simulink model "PD_Controller_mod"  (R2019b)
settings: Solver=VariableStepAuto  StartTime=0.0  StopTime=10  RelTol=1e-3
StopFcn:
  | Colors=hsv(5)';
  | for i=1:5
  | plot(out.tout,out.R_PD(:,i),'color',Colors(:,i),'LineWidth',1.5)
  | hold on
  | end
  | grid on
  | legend('Joint1','Joint2','Joint3','Joint4','Joint5')
  | title(['Response Vs Input of Joints Via PD Controller'])
  | xlabel('Time')
  | ylabel('Response')
libraries: simulink x5
(part 3 of 3)

== matlab function PD_Controller_mod/Robot_e_baba2 ==
  data: U input; q_ddot output; t input; tdot input
function q_ddot=fcn(U,t,tdot)

% t1=t(1);
t2=t(2);
t3=t(3);
t4=t(4);
t5=t(5);
% t6=t(6);

thetadot1=tdot(1);
thetadot2=tdot(2);
thetadot3=tdot(3);
thetadot4=tdot(4);
thetadot5=tdot(5);
% thetadot6=tdot(6);


M=[0.011148*cos(t5) + 4.3855*sin(t3) + 0.010268*cos(t5)*sin(t3) - 12.167*cos(t2)^2 - 1.6789*cos(t3)^2 - 0.0021796*cos(t4)^2 - 0.011148*cos(t2)^2*cos(t5) - 0.011148*cos(t3)^2*cos(t5) - 4.3855*cos(t2)^2*sin(t3) + 3.3578*cos(t2)^2*cos(t3)^2 + 0.0021796*cos(t2)^2*cos(t4)^2 - 0.00017962*cos(t2)^2*cos(t5)^2 + 0.0021796*cos(t3)^2*cos(t4)^2 - 0.00017962*cos(t3)^2*cos(t5)^2 + 0.00017962*cos(t4)^2*cos(t5)^2 - 0.0043592*cos(t2)^2*cos(t3)^2*cos(t4)^2 + 0.00035923*cos(t2)^2*cos(t3)^2*cos(t5)^2 - 0.00017962*cos(t2)^2*cos(t4)^2*cos(t5)^2 - 0.00017962*cos(t3)^2*cos(t4)^2*cos(t5)^2 - 0.010268*cos(t2)^2*cos(t5)*sin(t3) + 0.022296*cos(t2)^2*cos(t3)^2*cos(t5) - 4.3855*cos(t2)*cos(t3)*sin(t2) + 0.002*cos(t2)*cos(t4)*sin(t2) + 0.002*cos(t3)*cos(t4)*sin(t3) + 0.010268*cos(t3)*cos(t4)*sin(t5) - 0.004*cos(t2)*cos(t3)^2*cos(t4)*sin(t2) - 0.004*cos(t2)^2*cos(t3)*cos(t4)*sin(t3) - 0.010268*cos(t2)^2*cos(t3)*cos(t4)*sin(t5) + 0.00035923*cos(t2)^2*cos(t3)^2*cos(t4)^2*cos(t5)^2 - 0.010268*cos(t2)*cos(t3)*cos(t5)*sin(t2) - 3.3578*cos(t2)*cos(t3)*sin(t2)*sin(t3) + 0.011148*cos(t2)*cos(t4)*sin(t2)*sin(t5) + 0.011148*cos(t3)*cos(t4)*sin(t3)*sin(t5) + 0.0043592*cos(t2)*cos(t3)*cos(t4)^2*sin(t2)*sin(t3) - 0.00035923*cos(t2)*cos(t3)*cos(t5)^2*sin(t2)*sin(t3) - 0.022296*cos(t2)*cos(t3)^2*cos(t4)*sin(t2)*sin(t5) - 0.022296*cos(t2)^2*cos(t3)*cos(t4)*sin(t3)*sin(t5) - 0.022296*cos(t2)*cos(t3)*cos(t5)*sin(t2)*sin(t3) + 0.00035923*cos(t2)*cos(t4)*cos(t5)*sin(t2)*sin(t5) + 0.00035923*cos(t3)*cos(t4)*cos(t5)*sin(t3)*sin(t5) + 0.010268*cos(t2)*cos(t4)*sin(t2)*sin(t3)*sin(t5) - 0.00035923*cos(t2)*cos(t3)*cos(t4)^2*cos(t5)^2*sin(t2)*sin(t3) - 0.00071846*cos(t2)*cos(t3)^2*cos(t4)*cos(t5)*sin(t2)*sin(t5) - 0.00071846*cos(t2)^2*cos(t3)*cos(t4)*cos(t5)*sin(t3)*sin(t5) + 12.723, 0.11866*cos(t2) - 0.001*cos(t2)*cos(t3) + 0.001*sin(t2)*sin(t3) - 0.001*cos(t2)*sin(t3)*sin(t4) - 0.001*cos(t3)*sin(t2)*sin(t4) - 0.0051341*cos(t2)*sin(t4)*sin(t5) - 0.0021796*cos(t2)*cos(t3)*cos(t4)*sin(t4) + 0.0021796*cos(t4)*sin(t2)*sin(t3)*sin(t4) - 0.0055741*cos(t2)*sin(t3)*sin(t4)*sin(t5) - 0.0055741*cos(t3)*sin(t2)*sin(t4)*sin(t5) + 0.00017962*cos(t2)*cos(t3)*cos(t4)*cos(t5)^2*sin(t4) - 0.00017962*cos(t4)*cos(t5)^2*sin(t2)*sin(t3)*sin(t4) - 0.00017962*cos(t2)*cos(t5)*sin(t3)*sin(t4)*sin(t5) - 0.00017962*cos(t3)*cos(t5)*sin(t2)*sin(t4)*sin(t5), 0.001*sin(t2)*sin(t3) - 0.001*cos(t2)*cos(t3) - 0.001*cos(t2)*sin(t3)*sin(t4) - 0.001*cos(t3)*sin(t2)*sin(t4) - 0.0010449*sin(2.0*t4)*cos(t2)*cos(t3) + 0.0010449*sin(2.0*t4)*sin(t2)*sin(t3) + 0.000044904*cos(2.0*t5)*sin(2.0*t4)*cos(t2)*cos(t3) - 0.000044904*cos(2.0*t5)*sin(2.0*t4)*sin(t2)*sin(t3) - 0.000089808*sin(2.0*t5)*cos(t2)*sin(t3)*sin(t4) - 0.000089808*sin(2.0*t5)*cos(t3)*sin(t2)*sin(t4) - 0.0055741*cos(t2)*sin(t3)*sin(t4)*sin(t5) - 0.0055741*cos(t3)*sin(t2)*sin(t4)*sin(t5), 0.013*cos(t2)*sin(t3) + 0.013*cos(t3)*sin(t2) + 0.001*cos(t4)*sin(t2)*sin(t3) + 0.0051341*cos(t4)*sin(t2)*sin(t5) + 0.00017962*cos(t2)*sin(t3)*sin(t5)^2 + 0.00017962*cos(t3)*sin(t2)*sin(t5)^2 - 0.001*cos(t2)*cos(t3)*cos(t4) - 0.0055741*cos(t2)*cos(t3)*cos(t4)*sin(t5) + 0.0055741*cos(t4)*sin(t2)*sin(t3)*sin(t5) - 0.00017962*cos(t2)*cos(t3)*cos(t4)*cos(t5)*sin(t5) + 0.00017962*cos(t4)*cos(t5)*sin(t2)*sin(t3)*sin(t5), 1.0e-36*sin(t4)*(5.1341e+33*cos(t5)*sin(t2) - 1.7962e+32*cos(t2)*cos(t3) + 1.7962e+32*sin(t2)*sin(t3) + 5.5741e+33*cos(t5)*sin(t2)*sin(t3) - 5.5741e+33*cos(t2)*cos(t3)*cos(t5)), 0;
                                                                                                                                                                                                                                                                                                                                                                                                                                                                                                                                                                                                                                                                                                                                                                                                                                                                                                                                                                                                                                        0.11566*cos(t2) - 0.001*cos(t2)*cos(t3) + 0.001*sin(t2)*sin(t3) + 1.4349e-42*cos(2.0*t4)*cos(t2) - 0.001*cos(t2)*sin(t3)*sin(t4) - 0.001*cos(t3)*sin(t2)*sin(t4) - 0.0051341*cos(t2)*sin(t4)*sin(t5) + 3.5873e-43*cos(2.0*t3)*cos(2.0*t4)*cos(t2) + 3.5873e-43*cos(2.0*t4)*cos(2.0*t5)*cos(t2) + 3.5873e-43*cos(2.0*t4)*sin(2.0*t3)*sin(t2) - 3.5873e-43*cos(2.0*t5)*sin(2.0*t4)*sin(t2) - 0.0010449*sin(2.0*t4)*cos(t2)*cos(t3) + 0.0010449*sin(2.0*t4)*sin(t2)*sin(t3) + 0.000044904*cos(2.0*t5)*sin(2.0*t4)*cos(t2)*cos(t3) - 0.000044904*cos(2.0*t5)*sin(2.0*t4)*sin(t2)*sin(t3) - 0.000089808*sin(2.0*t5)*cos(t2)*sin(t3)*sin(t4) - 0.000089808*sin(2.0*t5)*cos(t3)*sin(t2)*sin(t4) - 0.0055741*cos(t2)*sin(t3)*sin(t4)*sin(t5) - 0.0055741*cos(t3)*sin(t2)*sin(t4)*sin(t5),                                                                                                                                                                                                                                                                                                                                                                                      0.011148*cos(t5) + 4.3855*sin(t3) + 0.010268*cos(t5)*sin(t3) + 0.0021796*cos(t4)^2 + 0.00017962*cos(t5)^2 - 0.00017962*cos(t4)^2*cos(t5)^2 + 0.010268*cos(t3)*cos(t4)*sin(t5) + 12.327,                                                                                                                                                                                                                                                                   0.0010449*cos(2.0*t4) + 0.000044904*cos(2.0*t5) + 0.011148*cos(t5) + 2.1928*sin(t3) + 0.0051341*cos(t5)*sin(t3) - 0.000044904*cos(2.0*t4)*cos(2.0*t5) + 1.5067e-40*cos(2.0*t4)*sin(t3) + 0.0051341*cos(t3)*cos(t4)*sin(t5) + 1.7641,                                                                                                                                                                                                                                                                                                                            -8.0e-36*sin(t4)*(1.1226e+31*sin(2.0*t5) + 6.9676e+32*sin(t5) + 6.4176e+32*sin(t3)*sin(t5) + 1.25e+32),                                                                   0.00017962*cos(t4) + 0.0055741*cos(t4)*cos(t5) + 0.0051341*cos(t3)*sin(t5) + 0.0051341*cos(t4)*cos(t5)*sin(t3), 0;
                                                                                                                                                                                                                                                                                                                                                                                                                                                                                                                                                                                                                                                                                                                                                                                                                                                                                                                                                                                                                                                                                                                                                                                                                                                                                                                   0.001*sin(t2)*sin(t3) - 0.001*cos(t2)*cos(t3) - 0.001*cos(t2)*sin(t3)*sin(t4) - 0.001*cos(t3)*sin(t2)*sin(t4) - 0.0010449*sin(2.0*t4)*cos(t2)*cos(t3) + 0.0010449*sin(2.0*t4)*sin(t2)*sin(t3) + 0.000044904*cos(2.0*t5)*sin(2.0*t4)*cos(t2)*cos(t3) - 0.000044904*cos(2.0*t5)*sin(2.0*t4)*sin(t2)*sin(t3) - 0.000089808*sin(2.0*t5)*cos(t2)*sin(t3)*sin(t4) - 0.000089808*sin(2.0*t5)*cos(t3)*sin(t2)*sin(t4) - 0.0055741*cos(t2)*sin(t3)*sin(t4)*sin(t5) - 0.0055741*cos(t3)*sin(t2)*sin(t4)*sin(t5),                                                                                                                                                                                                                                                                                                                                                                                    0.011148*cos(t5) + 2.1928*sin(t3) + 0.0051341*cos(t5)*sin(t3) + 0.0021796*cos(t4)^2 + 0.00017962*cos(t5)^2 - 0.00017962*cos(t4)^2*cos(t5)^2 + 0.0051341*cos(t3)*cos(t4)*sin(t5) + 1.7629,                                                                                                                                                                                                                                                                                                                                                                                     0.0010449*cos(2.0*t4) + 0.000044904*cos(2.0*t5) + 0.011148*cos(t5) - 0.000044904*cos(2.0*t4)*cos(2.0*t5) + 1.7641,                                                                                                                                                                                                                                                                                                                                                          -2.0e-36*sin(t4)*(4.4904e+31*sin(2.0*t5) + 2.7871e+33*sin(t5) + 5.0e+32),                                                                                                                                1.0e-36*cos(t4)*(5.5741e+33*cos(t5) + 1.7962e+32), 0;
                                                                                                                                                                                                                                                                                                                                                                                                                                                                                                                                                                                                                                                                                                                                                                                                                                                                                                                                                                                                                                                                                                                                                                                                                                                                                                                                                                                   0.01318*cos(t2)*sin(t3) + 0.01318*cos(t3)*sin(t2) + 0.001*cos(t4)*sin(t2)*sin(t3) + 0.0051341*cos(t4)*sin(t2)*sin(t5) - 0.00017962*cos(t2)*cos(t5)^2*sin(t3) - 0.00017962*cos(t3)*cos(t5)^2*sin(t2) - 0.001*cos(t2)*cos(t3)*cos(t4) - 0.0055741*cos(t2)*cos(t3)*cos(t4)*sin(t5) + 0.0055741*cos(t4)*sin(t2)*sin(t3)*sin(t5) - 0.00017962*cos(t2)*cos(t3)*cos(t4)*cos(t5)*sin(t5) + 0.00017962*cos(t4)*cos(t5)*sin(t2)*sin(t3)*sin(t5),                                                                                                                                                                                                                                                                                                                                                                                                                                                                      -8.0e-36*sin(t4)*(1.1226e+31*sin(2.0*t5) + 6.9676e+32*sin(t5) + 6.4176e+32*sin(t3)*sin(t5) + 1.25e+32),                                                                                                                                                                                                                                                                                                                                                                                                                             -8.0e-36*sin(t4)*(1.1226e+31*sin(2.0*t5) + 6.9676e+32*sin(t5) + 1.25e+32),                                                                                                                                                                                                                                                                                                                                                                                                      0.00017962*sin(t5)^2 + 0.013,                                                                                                                                                                                0, 0;
                                                                                                                                                                                                                                                                                                                                                                                                                                                                                                                                                                                                                                                                                                                                                                                                                                                                                                                                                                                                                                                                                                                                                                                                                                                                                                                                                                                                                                                                                                                                                                                                                                          2.4e-35*sin(t4)*(2.1392e+32*cos(t5)*sin(t2) - 7.484e+30*cos(t2)*cos(t3) + 7.484e+30*sin(t2)*sin(t3) + 2.3225e+32*cos(t5)*sin(t2)*sin(t3) - 2.3225e+32*cos(t2)*cos(t3)*cos(t5)),                                                                                                                                                                                                                                                                                                                                                                                                                                                              0.00017962*cos(t4) + 0.0055741*cos(t4)*cos(t5) + 0.0051341*cos(t3)*sin(t5) + 0.0051341*cos(t4)*cos(t5)*sin(t3),                                                                                                                                                                                                                                                                                                                                                                                                                                                      2.4e-35*cos(t4)*(2.3225e+32*cos(t5) + 7.484e+30),                                                                                                                                                                                                                                                                                                                                                                                                                                 0,                                                                                                                                                                       0.00017962, 0;
                                                                                                                                                                                                                                                                                                                                                                                                                                                                                                                                                                                                                                                                                                                                                                                                                                                                                                                                                                                                                                                                                                                                                                                                                                                                                                                                                                                                                                                                                                                                                                                                                                                                                                                                                                                                                       0,                                                                                                                                                                                                                                                                                                                                                                                                                                                                                                                                                                           0,                                                                                                                                                                                                                                                                                                                                                                                                                                                                                                     0,                                                                                                                                                                                                                                                                                                                                                                                                                                 0,                                                                                                                                                                                0, 0];




                                                                                                                                                                                                                                                                                                                                                                                                                                                                                                                                                                                                                                                                                                                                                                                                                                                                                                                                                                                                                                                                                                                                                                                                                                                                                                                                                                                                                                                                                                                                                                                                                                                                                                                                                                                                                   


C=[10.488*thetadot2*sin(2.0*t2) + 0.0010449*thetadot4*sin(2.0*t4) + 0.000044904*thetadot5*sin(2.0*t5) + 2.1928*thetadot3*cos(t3) - 0.0055741*thetadot5*sin(t5) - 4.3855*thetadot2*cos(2.0*t2)*cos(t3) - 2.1928*thetadot3*cos(2.0*t2)*cos(t3) + 4.3855*thetadot2*sin(2.0*t2)*sin(t3) + 2.1928*thetadot3*sin(2.0*t2)*sin(t3) + 0.0051341*thetadot3*cos(t3)*cos(t5) - 0.0051341*thetadot5*sin(t3)*sin(t5) - 1.678*thetadot2*cos(2.0*t2)*sin(2.0*t3) - 1.678*thetadot2*cos(2.0*t3)*sin(2.0*t2) - 1.678*thetadot3*cos(2.0*t2)*sin(2.0*t3) - 1.678*thetadot3*cos(2.0*t3)*sin(2.0*t2) - 0.000044904*thetadot4*cos(2.0*t5)*sin(2.0*t4) - 0.000044904*thetadot5*cos(2.0*t4)*sin(2.0*t5) + 0.010268*thetadot2*sin(2.0*t2)*cos(t5)*sin(t3) + 0.0051341*thetadot3*sin(2.0*t2)*cos(t5)*sin(t3) + 0.0051341*thetadot5*cos(2.0*t2)*sin(t3)*sin(t5) + 0.0051341*thetadot5*sin(2.0*t2)*cos(t3)*sin(t5) + 0.0010449*thetadot2*cos(2.0*t2)*cos(2.0*t4)*sin(2.0*t3) + 0.0010449*thetadot2*cos(2.0*t3)*cos(2.0*t4)*sin(2.0*t2) - 0.00013471*thetadot2*cos(2.0*t2)*cos(2.0*t5)*sin(2.0*t3) - 0.00013471*thetadot2*cos(2.0*t3)*cos(2.0*t5)*sin(2.0*t2) + 0.0010449*thetadot3*cos(2.0*t2)*cos(2.0*t4)*sin(2.0*t3) + 0.0010449*thetadot3*cos(2.0*t3)*cos(2.0*t4)*sin(2.0*t2) - 0.00013471*thetadot3*cos(2.0*t2)*cos(2.0*t5)*sin(2.0*t3) - 0.00013471*thetadot3*cos(2.0*t3)*cos(2.0*t5)*sin(2.0*t2) + 0.0010449*thetadot4*cos(2.0*t2)*cos(2.0*t3)*sin(2.0*t4) - 0.00013471*thetadot5*cos(2.0*t2)*cos(2.0*t3)*sin(2.0*t5) + 0.0051341*thetadot5*cos(t3)*cos(t4)*cos(t5) - 0.0010449*thetadot4*sin(2.0*t2)*sin(2.0*t3)*sin(2.0*t4) + 0.00013471*thetadot5*sin(2.0*t2)*sin(2.0*t3)*sin(2.0*t5) - 0.0051341*thetadot3*cos(t4)*sin(t3)*sin(t5) - 0.0051341*thetadot4*cos(t3)*sin(t4)*sin(t5) - 0.002*thetadot2*cos(2.0*t2)*cos(2.0*t3)*cos(t4) - 0.002*thetadot3*cos(2.0*t2)*cos(2.0*t3)*cos(t4) - 0.011148*thetadot2*cos(2.0*t2)*sin(2.0*t3)*cos(t5) - 0.011148*thetadot2*cos(2.0*t3)*sin(2.0*t2)*cos(t5) - 0.011148*thetadot3*cos(2.0*t2)*sin(2.0*t3)*cos(t5) - 0.011148*thetadot3*cos(2.0*t3)*sin(2.0*t2)*cos(t5) - 0.0055741*thetadot5*cos(2.0*t2)*cos(2.0*t3)*sin(t5) + 0.002*thetadot2*sin(2.0*t2)*sin(2.0*t3)*cos(t4) + 0.002*thetadot3*sin(2.0*t2)*sin(2.0*t3)*cos(t4) + 0.001*thetadot4*cos(2.0*t2)*sin(2.0*t3)*sin(t4) + 0.001*thetadot4*cos(2.0*t3)*sin(2.0*t2)*sin(t4) + 0.0055741*thetadot5*sin(2.0*t2)*sin(2.0*t3)*sin(t5) - 0.010268*thetadot2*cos(2.0*t2)*cos(t3)*cos(t5) - 0.0051341*thetadot3*cos(2.0*t2)*cos(t3)*cos(t5) - 0.0051341*thetadot4*sin(2.0*t2)*sin(t3)*sin(t4)*sin(t5) - 0.00017962*thetadot2*cos(2.0*t2)*cos(2.0*t3)*sin(2.0*t5)*cos(t4) - 0.00017962*thetadot3*cos(2.0*t2)*cos(2.0*t3)*sin(2.0*t5)*cos(t4) - 0.00017962*thetadot5*cos(2.0*t2)*cos(2.0*t5)*sin(2.0*t3)*cos(t4) - 0.00017962*thetadot5*cos(2.0*t3)*cos(2.0*t5)*sin(2.0*t2)*cos(t4) + 0.00017962*thetadot2*sin(2.0*t2)*sin(2.0*t3)*sin(2.0*t5)*cos(t4) + 0.00017962*thetadot3*sin(2.0*t2)*sin(2.0*t3)*sin(2.0*t5)*cos(t4) + 0.000089808*thetadot4*cos(2.0*t2)*sin(2.0*t3)*sin(2.0*t5)*sin(t4) + 0.000089808*thetadot4*cos(2.0*t3)*sin(2.0*t2)*sin(2.0*t5)*sin(t4) - 0.011148*thetadot2*cos(2.0*t2)*cos(2.0*t3)*cos(t4)*sin(t5) - 0.011148*thetadot3*cos(2.0*t2)*cos(2.0*t3)*cos(t4)*sin(t5) - 0.0055741*thetadot5*cos(2.0*t2)*sin(2.0*t3)*cos(t4)*cos(t5) - 0.0055741*thetadot5*cos(2.0*t3)*sin(2.0*t2)*cos(t4)*cos(t5) + 0.011148*thetadot2*sin(2.0*t2)*sin(2.0*t3)*cos(t4)*sin(t5) + 0.011148*thetadot3*sin(2.0*t2)*sin(2.0*t3)*cos(t4)*sin(t5) + 0.0055741*thetadot4*cos(2.0*t2)*sin(2.0*t3)*sin(t4)*sin(t5) + 0.0055741*thetadot4*cos(2.0*t3)*sin(2.0*t2)*sin(t4)*sin(t5) - 0.000044904*thetadot2*cos(2.0*t2)*cos(2.0*t4)*cos(2.0*t5)*sin(2.0*t3) - 0.000044904*thetadot2*cos(2.0*t3)*cos(2.0*t4)*cos(2.0*t5)*sin(2.0*t2) - 0.000044904*thetadot3*cos(2.0*t2)*cos(2.0*t4)*cos(2.0*t5)*sin(2.0*t3) - 0.000044904*thetadot3*cos(2.0*t3)*cos(2.0*t4)*cos(2.0*t5)*sin(2.0*t2) - 0.000044904*thetadot4*cos(2.0*t2)*cos(2.0*t3)*cos(2.0*t5)*sin(2.0*t4) - 0.000044904*thetadot5*cos(2.0*t2)*cos(2.0*t3)*cos(2.0*t4)*sin(2.0*t5) - 0.0051341*thetadot5*cos(2.0*t2)*cos(t3)*cos(t4)*cos(t5) + 0.000044904*thetadot4*cos(2.0*t5)*sin(2.0*t2)*sin(2.0*t3)*sin(2.0*t4) + 0.000044904*thetadot5*cos(2.0*t4)*sin(2.0*t2)*sin(2.0*t3)*sin(2.0*t5) + 0.010268*thetadot2*cos(2.0*t2)*cos(t4)*sin(t3)*sin(t5) + 0.010268*thetadot2*sin(2.0*t2)*cos(t3)*cos(t4)*sin(t5) + 0.0051341*thetadot3*cos(2.0*t2)*cos(t4)*sin(t3)*sin(t5) + 0.0051341*thetadot3*sin(2.0*t2)*cos(t3)*cos(t4)*sin(t5) + 0.0051341*thetadot4*cos(2.0*t2)*cos(t3)*sin(t4)*sin(t5) + 0.0051341*thetadot5*sin(2.0*t2)*cos(t4)*cos(t5)*sin(t3), 10.488*thetadot1*sin(2.0*t2) - 0.11866*thetadot2*sin(t2) - 4.3855*thetadot1*cos(2.0*t2)*cos(t3) + 4.3855*thetadot1*sin(2.0*t2)*sin(t3) + 0.01309*thetadot4*cos(t2)*cos(t3) + 0.001*thetadot2*cos(t2)*sin(t3) + 0.001*thetadot2*cos(t3)*sin(t2) + 0.002*thetadot3*cos(t2)*sin(t3) + 0.002*thetadot3*cos(t3)*sin(t2) - 0.01309*thetadot4*sin(t2)*sin(t3) - 1.678*thetadot1*cos(2.0*t2)*sin(2.0*t3) - 1.678*thetadot1*cos(2.0*t3)*sin(2.0*t2) + 0.010268*thetadot1*sin(2.0*t2)*cos(t5)*sin(t3) + 0.0010449*thetadot2*sin(2.0*t4)*cos(t2)*sin(t3) + 0.0010449*thetadot2*sin(2.0*t4)*cos(t3)*sin(t2) + 0.0020898*thetadot3*sin(2.0*t4)*cos(t2)*sin(t3) + 0.0020898*thetadot3*sin(2.0*t4)*cos(t3)*sin(t2) + 0.0020898*thetadot4*cos(2.0*t4)*sin(t2)*sin(t3) + 0.000089808*thetadot4*cos(2.0*t5)*sin(t2)*sin(t3) + 0.0010449*thetadot1*cos(2.0*t2)*cos(2.0*t4)*sin(2.0*t3) + 0.0010449*thetadot1*cos(2.0*t3)*cos(2.0*t4)*sin(2.0*t2) - 0.00013471*thetadot1*cos(2.0*t2)*cos(2.0*t5)*sin(2.0*t3) - 0.00013471*thetadot1*cos(2.0*t3)*cos(2.0*t5)*sin(2.0*t2) - 0.001*thetadot2*cos(t2)*cos(t3)*sin(t4) - 0.002*thetadot3*cos(t2)*cos(t3)*sin(t4) + 0.00017962*thetadot5*cos(t2)*sin(t3)*sin(t4) + 0.00017962*thetadot5*cos(t3)*sin(t2)*sin(t4) + 0.001*thetadot2*sin(t2)*sin(t3)*sin(t4) + 0.002*thetadot3*sin(t2)*sin(t3)*sin(t4) + 0.0051341*thetadot2*sin(t2)*sin(t4)*sin(t5) - 0.002*thetadot1*cos(2.0*t2)*cos(2.0*t3)*cos(t4) - 0.011148*thetadot1*cos(2.0*t2)*sin(2.0*t3)*cos(t5) - 0.011148*thetadot1*cos(2.0*t3)*sin(2.0*t2)*cos(t5) + 0.002*thetadot1*sin(2.0*t2)*sin(2.0*t3)*cos(t4) - 0.010268*thetadot1*cos(2.0*t2)*cos(t3)*cos(t5) - 0.0020898*thetadot4*cos(2.0*t4)*cos(t2)*cos(t3) - 0.000089808*thetadot4*cos(2.0*t5)*cos(t2)*cos(t3) + 0.000089808*thetadot2*sin(2.0*t5)*sin(t2)*sin(t3)*sin(t4) + 0.00017962*thetadot3*sin(2.0*t5)*sin(t2)*sin(t3)*sin(t4) - 0.00017962*thetadot1*cos(2.0*t2)*cos(2.0*t3)*sin(2.0*t5)*cos(t4) + 0.00017962*thetadot1*sin(2.0*t2)*sin(2.0*t3)*sin(2.0*t5)*cos(t4) - 0.0055741*thetadot2*cos(t2)*cos(t3)*sin(t4)*sin(t5) - 0.011148*thetadot3*cos(t2)*cos(t3)*sin(t4)*sin(t5) + 0.000089808*thetadot4*cos(2.0*t4)*cos(2.0*t5)*cos(t2)*cos(t3) + 0.0055741*thetadot2*sin(t2)*sin(t3)*sin(t4)*sin(t5) + 0.011148*thetadot3*sin(t2)*sin(t3)*sin(t4)*sin(t5) - 0.011148*thetadot1*cos(2.0*t2)*cos(2.0*t3)*cos(t4)*sin(t5) - 0.000044904*thetadot2*cos(2.0*t5)*sin(2.0*t4)*cos(t2)*sin(t3) - 0.000044904*thetadot2*cos(2.0*t5)*sin(2.0*t4)*cos(t3)*sin(t2) - 0.000089808*thetadot3*cos(2.0*t5)*sin(2.0*t4)*cos(t2)*sin(t3) - 0.000089808*thetadot3*cos(2.0*t5)*sin(2.0*t4)*cos(t3)*sin(t2) - 0.000089808*thetadot4*cos(2.0*t4)*cos(2.0*t5)*sin(t2)*sin(t3) - 0.000089808*thetadot5*sin(2.0*t4)*sin(2.0*t5)*cos(t2)*cos(t3) + 0.011148*thetadot1*sin(2.0*t2)*sin(2.0*t3)*cos(t4)*sin(t5) + 0.000089808*thetadot5*sin(2.0*t4)*sin(2.0*t5)*sin(t2)*sin(t3) - 0.000044904*thetadot1*cos(2.0*t2)*cos(2.0*t4)*cos(2.0*t5)*sin(2.0*t3) - 0.000044904*thetadot1*cos(2.0*t3)*cos(2.0*t4)*cos(2.0*t5)*sin(2.0*t2) + 0.010268*thetadot1*cos(2.0*t2)*cos(t4)*sin(t3)*sin(t5) + 0.010268*thetadot1*sin(2.0*t2)*cos(t3)*cos(t4)*sin(t5) - 0.000089808*thetadot2*sin(2.0*t5)*cos(t2)*cos(t3)*sin(t4) - 0.00017962*thetadot3*sin(2.0*t5)*cos(t2)*cos(t3)*sin(t4) - 0.00017962*thetadot5*cos(2.0*t5)*cos(t2)*sin(t3)*sin(t4) - 0.00017962*thetadot5*cos(2.0*t5)*cos(t3)*sin(t2)*sin(t4), 2.1928*thetadot1*cos(t3) - 2.1928*thetadot1*cos(2.0*t2)*cos(t3) + 2.1928*thetadot1*sin(2.0*t2)*sin(t3) + 0.0051341*thetadot1*cos(t3)*cos(t5) + 0.01309*thetadot4*cos(t2)*cos(t3) + 0.002*thetadot2*cos(t2)*sin(t3) + 0.002*thetadot2*cos(t3)*sin(t2) + 0.001*thetadot3*cos(t2)*sin(t3) + 0.001*thetadot3*cos(t3)*sin(t2) - 0.01309*thetadot4*sin(t2)*sin(t3) - 1.678*thetadot1*cos(2.0*t2)*sin(2.0*t3) - 1.678*thetadot1*cos(2.0*t3)*sin(2.0*t2) + 0.0051341*thetadot1*sin(2.0*t2)*cos(t5)*sin(t3) + 0.0020898*thetadot2*sin(2.0*t4)*cos(t2)*sin(t3) + 0.0020898*thetadot2*sin(2.0*t4)*cos(t3)*sin(t2) + 0.0010449*thetadot3*sin(2.0*t4)*cos(t2)*sin(t3) + 0.0010449*thetadot3*sin(2.0*t4)*cos(t3)*sin(t2) + 0.0020898*thetadot4*cos(2.0*t4)*sin(t2)*sin(t3) + 0.000089808*thetadot4*cos(2.0*t5)*sin(t2)*sin(t3) + 0.0010449*thetadot1*cos(2.0*t2)*cos(2.0*t4)*sin(2.0*t3) + 0.0010449*thetadot1*cos(2.0*t3)*cos(2.0*t4)*sin(2.0*t2) - 0.00013471*thetadot1*cos(2.0*t2)*cos(2.0*t5)*sin(2.0*t3) - 0.00013471*thetadot1*cos(2.0*t3)*cos(2.0*t5)*sin(2.0*t2) - 0.002*thetadot2*cos(t2)*cos(t3)*sin(t4) - 0.001*thetadot3*cos(t2)*cos(t3)*sin(t4) - 0.0051341*thetadot1*cos(t4)*sin(t3)*sin(t5) + 0.00017962*thetadot5*cos(t2)*sin(t3)*sin(t4) + 0.00017962*thetadot5*cos(t3)*sin(t2)*sin(t4) + 0.002*thetadot2*sin(t2)*sin(t3)*sin(t4) + 0.001*thetadot3*sin(t2)*sin(t3)*sin(t4) - 0.002*thetadot1*cos(2.0*t2)*cos(2.0*t3)*cos(t4) - 0.011148*thetadot1*cos(2.0*t2)*sin(2.0*t3)*cos(t5) - 0.011148*thetadot1*cos(2.0*t3)*sin(2.0*t2)*cos(t5) + 0.002*thetadot1*sin(2.0*t2)*sin(2.0*t3)*cos(t4) - 0.0051341*thetadot1*cos(2.0*t2)*cos(t3)*cos(t5) - 0.0020898*thetadot4*cos(2.0*t4)*cos(t2)*cos(t3) - 0.000089808*thetadot4*cos(2.0*t5)*cos(t2)*cos(t3) + 0.00017962*thetadot2*sin(2.0*t5)*sin(t2)*sin(t3)*sin(t4) + 0.000089808*thetadot3*sin(2.0*t5)*sin(t2)*sin(t3)*sin(t4) - 0.00017962*thetadot1*cos(2.0*t2)*cos(2.0*t3)*sin(2.0*t5)*cos(t4) + 0.00017962*thetadot1*sin(2.0*t2)*sin(2.0*t3)*sin(2.0*t5)*cos(t4) - 0.011148*thetadot2*cos(t2)*cos(t3)*sin(t4)*sin(t5) - 0.0055741*thetadot3*cos(t2)*cos(t3)*sin(t4)*sin(t5) + 0.000089808*thetadot4*cos(2.0*t4)*cos(2.0*t5)*cos(t2)*cos(t3) + 0.011148*thetadot2*sin(t2)*sin(t3)*sin(t4)*sin(t5) + 0.0055741*thetadot3*sin(t2)*sin(t3)*sin(t4)*sin(t5) - 0.011148*thetadot1*cos(2.0*t2)*cos(2.0*t3)*cos(t4)*sin(t5) - 0.000089808*thetadot2*cos(2.0*t5)*sin(2.0*t4)*cos(t2)*sin(t3) - 0.000089808*thetadot2*cos(2.0*t5)*sin(2.0*t4)*cos(t3)*sin(t2) - 0.000044904*thetadot3*cos(2.0*t5)*sin(2.0*t4)*cos(t2)*sin(t3) - 0.000044904*thetadot3*cos(2.0*t5)*sin(2.0*t4)*cos(t3)*sin(t2) - 0.000089808*thetadot4*cos(2.0*t4)*cos(2.0*t5)*sin(t2)*sin(t3) - 0.000089808*thetadot5*sin(2.0*t4)*sin(2.0*t5)*cos(t2)*cos(t3) + 0.011148*thetadot1*sin(2.0*t2)*sin(2.0*t3)*cos(t4)*sin(t5) + 0.000089808*thetadot5*sin(2.0*t4)*sin(2.0*t5)*sin(t2)*sin(t3) - 0.000044904*thetadot1*cos(2.0*t2)*cos(2.0*t4)*cos(2.0*t5)*sin(2.0*t3) - 0.000044904*thetadot1*cos(2.0*t3)*cos(2.0*t4)*cos(2.0*t5)*sin(2.0*t2) + 0.0051341*thetadot1*cos(2.0*t2)*cos(t4)*sin(t3)*sin(t5) + 0.0051341*thetadot1*sin(2.0*t2)*cos(t3)*cos(t4)*sin(t5) - 0.00017962*thetadot2*sin(2.0*t5)*cos(t2)*cos(t3)*sin(t4) - 0.000089808*thetadot3*sin(2.0*t5)*cos(t2)*cos(t3)*sin(t4) - 0.00017962*thetadot5*cos(2.0*t5)*cos(t2)*sin(t3)*sin(t4) - 0.00017962*thetadot5*cos(2.0*t5)*cos(t3)*sin(t2)*sin(t4), 0.0010449*thetadot1*sin(2.0*t4) + 0.01309*thetadot2*cos(t2)*cos(t3) + 0.01309*thetadot3*cos(t2)*cos(t3) - 0.01309*thetadot2*sin(t2)*sin(t3) - 0.01309*thetadot3*sin(t2)*sin(t3) - 0.000044904*thetadot1*cos(2.0*t5)*sin(2.0*t4) + 0.0020898*thetadot2*cos(2.0*t4)*sin(t2)*sin(t3) + 0.000089808*thetadot2*cos(2.0*t5)*sin(t2)*sin(t3) + 0.0020898*thetadot3*cos(2.0*t4)*sin(t2)*sin(t3) + 0.000089808*thetadot3*cos(2.0*t5)*sin(t2)*sin(t3) + 0.00017962*thetadot5*sin(2.0*t5)*cos(t2)*sin(t3) + 0.00017962*thetadot5*sin(2.0*t5)*cos(t3)*sin(t2) + 0.0010449*thetadot1*cos(2.0*t2)*cos(2.0*t3)*sin(2.0*t4) - 0.00017962*thetadot5*cos(t2)*cos(t3)*cos(t4) - 0.0010449*thetadot1*sin(2.0*t2)*sin(2.0*t3)*sin(2.0*t4) + 0.001*thetadot4*cos(t2)*cos(t3)*sin(t4) + 0.010268*thetadot5*cos(t4)*cos(t5)*sin(t2) - 0.0051341*thetadot1*cos(t3)*sin(t4)*sin(t5) + 0.00017962*thetadot5*cos(t4)*sin(t2)*sin(t3) - 0.001*thetadot4*sin(t2)*sin(t3)*sin(t4) - 0.0051341*thetadot4*sin(t2)*sin(t4)*sin(t5) + 0.001*thetadot1*cos(2.0*t2)*sin(2.0*t3)*sin(t4) + 0.001*thetadot1*cos(2.0*t3)*sin(2.0*t2)*sin(t4) - 0.0020898*thetadot2*cos(2.0*t4)*cos(t2)*cos(t3) - 0.000089808*thetadot2*cos(2.0*t5)*cos(t2)*cos(t3) - 0.0020898*thetadot3*cos(2.0*t4)*cos(t2)*cos(t3) - 0.000089808*thetadot3*cos(2.0*t5)*cos(t2)*cos(t3) - 0.0051341*thetadot1*sin(2.0*t2)*sin(t3)*sin(t4)*sin(t5) - 0.000089808*thetadot4*sin(2.0*t5)*sin(t2)*sin(t3)*sin(t4) - 0.011148*thetadot5*cos(t2)*cos(t3)*cos(t4)*cos(t5) + 0.000089808*thetadot1*cos(2.0*t2)*sin(2.0*t3)*sin(2.0*t5)*sin(t4) + 0.000089808*thetadot1*cos(2.0*t3)*sin(2.0*t2)*sin(2.0*t5)*sin(t4) + 0.0055741*thetadot4*cos(t2)*cos(t3)*sin(t4)*sin(t5) + 0.011148*thetadot5*cos(t4)*cos(t5)*sin(t2)*sin(t3) + 0.000089808*thetadot2*cos(2.0*t4)*cos(2.0*t5)*cos(t2)*cos(t3) + 0.000089808*thetadot3*cos(2.0*t4)*cos(2.0*t5)*cos(t2)*cos(t3) - 0.0055741*thetadot4*sin(t2)*sin(t3)*sin(t4)*sin(t5) - 0.000089808*thetadot2*cos(2.0*t4)*cos(2.0*t5)*sin(t2)*sin(t3) - 0.000089808*thetadot3*cos(2.0*t4)*cos(2.0*t5)*sin(t2)*sin(t3) + 0.0055741*thetadot1*cos(2.0*t2)*sin(2.0*t3)*sin(t4)*sin(t5) + 0.0055741*thetadot1*cos(2.0*t3)*sin(2.0*t2)*sin(t4)*sin(t5) - 0.000044904*thetadot1*cos(2.0*t2)*cos(2.0*t3)*cos(2.0*t5)*sin(2.0*t4) - 0.00017962*thetadot5*cos(2.0*t5)*cos(t2)*cos(t3)*cos(t4) + 0.000044904*thetadot1*cos(2.0*t5)*sin(2.0*t2)*sin(2.0*t3)*sin(2.0*t4) + 0.0051341*thetadot1*cos(2.0*t2)*cos(t3)*sin(t4)*sin(t5) + 0.000089808*thetadot4*sin(2.0*t5)*cos(t2)*cos(t3)*sin(t4) + 0.00017962*thetadot5*cos(2.0*t5)*cos(t4)*sin(t2)*sin(t3), 0.000044904*thetadot1*sin(2.0*t5) - 0.0055741*thetadot1*sin(t5) - 0.0051341*thetadot1*sin(t3)*sin(t5) - 0.000044904*thetadot1*cos(2.0*t4)*sin(2.0*t5) + 0.0051341*thetadot1*cos(2.0*t2)*sin(t3)*sin(t5) + 0.0051341*thetadot1*sin(2.0*t2)*cos(t3)*sin(t5) + 0.00017962*thetadot4*sin(2.0*t5)*cos(t2)*sin(t3) + 0.00017962*thetadot4*sin(2.0*t5)*cos(t3)*sin(t2) - 0.00013471*thetadot1*cos(2.0*t2)*cos(2.0*t3)*sin(2.0*t5) + 0.0051341*thetadot1*cos(t3)*cos(t4)*cos(t5) - 0.00017962*thetadot4*cos(t2)*cos(t3)*cos(t4) + 0.00013471*thetadot1*sin(2.0*t2)*sin(2.0*t3)*sin(2.0*t5) + 0.010268*thetadot4*cos(t4)*cos(t5)*sin(t2) + 0.00017962*thetadot2*cos(t2)*sin(t3)*sin(t4) + 0.00017962*thetadot2*cos(t3)*sin(t2)*sin(t4) + 0.00017962*thetadot3*cos(t2)*sin(t3)*sin(t4) + 0.00017962*thetadot3*cos(t3)*sin(t2)*sin(t4) + 0.00017962*thetadot4*cos(t4)*sin(t2)*sin(t3) - 0.0051341*thetadot5*sin(t2)*sin(t4)*sin(t5) - 0.0055741*thetadot1*cos(2.0*t2)*cos(2.0*t3)*sin(t5) + 0.0055741*thetadot1*sin(2.0*t2)*sin(2.0*t3)*sin(t5) - 0.00017962*thetadot1*cos(2.0*t2)*cos(2.0*t5)*sin(2.0*t3)*cos(t4) - 0.00017962*thetadot1*cos(2.0*t3)*cos(2.0*t5)*sin(2.0*t2)*cos(t4) - 0.011148*thetadot4*cos(t2)*cos(t3)*cos(t4)*cos(t5) + 0.011148*thetadot4*cos(t4)*cos(t5)*sin(t2)*sin(t3) + 0.0055741*thetadot5*cos(t2)*cos(t3)*sin(t4)*sin(t5) - 0.0055741*thetadot5*sin(t2)*sin(t3)*sin(t4)*sin(t5) - 0.0055741*thetadot1*cos(2.0*t2)*sin(2.0*t3)*cos(t4)*cos(t5) - 0.0055741*thetadot1*cos(2.0*t3)*sin(2.0*t2)*cos(t4)*cos(t5) - 0.000089808*thetadot2*sin(2.0*t4)*sin(2.0*t5)*cos(t2)*cos(t3) - 0.000089808*thetadot3*sin(2.0*t4)*sin(2.0*t5)*cos(t2)*cos(t3) + 0.000089808*thetadot2*sin(2.0*t4)*sin(2.0*t5)*sin(t2)*sin(t3) + 0.000089808*thetadot3*sin(2.0*t4)*sin(2.0*t5)*sin(t2)*sin(t3) - 0.000044904*thetadot1*cos(2.0*t2)*cos(2.0*t3)*cos(2.0*t4)*sin(2.0*t5) - 0.0051341*thetadot1*cos(2.0*t2)*cos(t3)*cos(t4)*cos(t5) - 0.00017962*thetadot4*cos(2.0*t5)*cos(t2)*cos(t3)*cos(t4) + 0.000044904*thetadot1*cos(2.0*t4)*sin(2.0*t2)*sin(2.0*t3)*sin(2.0*t5) + 0.0051341*thetadot1*sin(2.0*t2)*cos(t4)*cos(t5)*sin(t3) - 0.00017962*thetadot2*cos(2.0*t5)*cos(t2)*sin(t3)*sin(t4) - 0.00017962*thetadot2*cos(2.0*t5)*cos(t3)*sin(t2)*sin(t4) - 0.00017962*thetadot3*cos(2.0*t5)*cos(t2)*sin(t3)*sin(t4) - 0.00017962*thetadot3*cos(2.0*t5)*cos(t3)*sin(t2)*sin(t4) + 0.00017962*thetadot4*cos(2.0*t5)*cos(t4)*sin(t2)*sin(t3), 0;
                                                                                                                                                                                                                                                                                                                                                                                                                                                                                                                                                                                                                                                                                                                                                                                                                                                                                                                                                                                                                                                                                                                                                                                                                                                                                                                                                                                                                                                                                                                                                                                                                                                                                                                                                                                                                                                                                                                                                                                                                        0.003*thetadot2*sin(t2) - 5.2441*thetadot1*sin(2.0*t2) + 2.1928*thetadot1*cos(2.0*t2)*cos(t3) - 2.1928*thetadot1*sin(2.0*t2)*sin(t3) - 0.01309*thetadot4*cos(t2)*cos(t3) + 0.01309*thetadot4*sin(t2)*sin(t3) + 0.83898*thetadot1*cos(2.0*t2)*sin(2.0*t3) + 0.83898*thetadot1*cos(2.0*t3)*sin(2.0*t2) - 0.0051341*thetadot1*sin(2.0*t2)*cos(t5)*sin(t3) + 0.0020898*thetadot4*cos(2.0*t4)*sin(t2)*sin(t3) - 0.000089808*thetadot4*cos(2.0*t5)*sin(t2)*sin(t3) - 0.00052245*thetadot1*cos(2.0*t2)*cos(2.0*t4)*sin(2.0*t3) - 0.00052245*thetadot1*cos(2.0*t3)*cos(2.0*t4)*sin(2.0*t2) + 0.000067356*thetadot1*cos(2.0*t2)*cos(2.0*t5)*sin(2.0*t3) + 0.000067356*thetadot1*cos(2.0*t3)*cos(2.0*t5)*sin(2.0*t2) - 0.002*thetadot4*cos(t2)*cos(t4)*sin(t3) - 0.002*thetadot4*cos(t3)*cos(t4)*sin(t2) - 0.010268*thetadot4*cos(t2)*cos(t4)*sin(t5) - 0.010268*thetadot5*cos(t2)*cos(t5)*sin(t4) - 0.00017962*thetadot5*cos(t2)*sin(t3)*sin(t4) - 0.00017962*thetadot5*cos(t3)*sin(t2)*sin(t4) + 0.001*thetadot1*cos(2.0*t2)*cos(2.0*t3)*cos(t4) + 0.0055741*thetadot1*cos(2.0*t2)*sin(2.0*t3)*cos(t5) + 0.0055741*thetadot1*cos(2.0*t3)*sin(2.0*t2)*cos(t5) - 0.001*thetadot1*sin(2.0*t2)*sin(2.0*t3)*cos(t4) + 0.0051341*thetadot1*cos(2.0*t2)*cos(t3)*cos(t5) - 0.0020898*thetadot4*cos(2.0*t4)*cos(t2)*cos(t3) + 0.000089808*thetadot4*cos(2.0*t5)*cos(t2)*cos(t3) + 0.000089808*thetadot1*cos(2.0*t2)*cos(2.0*t3)*sin(2.0*t5)*cos(t4) - 0.000089808*thetadot1*sin(2.0*t2)*sin(2.0*t3)*sin(2.0*t5)*cos(t4) - 0.011148*thetadot4*cos(t2)*cos(t4)*sin(t3)*sin(t5) - 0.011148*thetadot4*cos(t3)*cos(t4)*sin(t2)*sin(t5) - 0.011148*thetadot5*cos(t2)*cos(t5)*sin(t3)*sin(t4) - 0.011148*thetadot5*cos(t3)*cos(t5)*sin(t2)*sin(t4) + 0.000089808*thetadot4*cos(2.0*t4)*cos(2.0*t5)*cos(t2)*cos(t3) + 0.0055741*thetadot1*cos(2.0*t2)*cos(2.0*t3)*cos(t4)*sin(t5) - 0.000089808*thetadot4*cos(2.0*t4)*cos(2.0*t5)*sin(t2)*sin(t3) - 0.000089808*thetadot5*sin(2.0*t4)*sin(2.0*t5)*cos(t2)*cos(t3) - 0.0055741*thetadot1*sin(2.0*t2)*sin(2.0*t3)*cos(t4)*sin(t5) + 0.000089808*thetadot5*sin(2.0*t4)*sin(2.0*t5)*sin(t2)*sin(t3) + 0.000022452*thetadot1*cos(2.0*t2)*cos(2.0*t4)*cos(2.0*t5)*sin(2.0*t3) + 0.000022452*thetadot1*cos(2.0*t3)*cos(2.0*t4)*cos(2.0*t5)*sin(2.0*t2) - 0.0051341*thetadot1*cos(2.0*t2)*cos(t4)*sin(t3)*sin(t5) - 0.0051341*thetadot1*sin(2.0*t2)*cos(t3)*cos(t4)*sin(t5) - 0.00017962*thetadot4*sin(2.0*t5)*cos(t2)*cos(t4)*sin(t3) - 0.00017962*thetadot4*sin(2.0*t5)*cos(t3)*cos(t4)*sin(t2) - 0.00017962*thetadot5*cos(2.0*t5)*cos(t2)*sin(t3)*sin(t4) - 0.00017962*thetadot5*cos(2.0*t5)*cos(t3)*sin(t2)*sin(t4),                                                                                                                                                                                                                                                                                                                                                                                                                                                                                                                                                                                                                                                                                                                                                                                                                                                                                                                                                                                                                                                                                                                                                                                                                                                                                                                                                                                                                                                                                                                                                                                                                                                                                                                                                                                                                                                                                                                                                                                                                                                                                                                                                                                                                                                                                                                                                                                                                                                                                                                                                                                                                                                                                                                                                                                                                                                                                                                                   4.3855*thetadot3*cos(t3) - 0.000089808*thetadot5*sin(2.0*t5) - 0.0020898*thetadot4*sin(2.0*t4) + 0.003*thetadot1*sin(t2) - 0.011148*thetadot5*sin(t5) + 0.010268*thetadot3*cos(t3)*cos(t5) - 0.010268*thetadot5*sin(t3)*sin(t5) + 0.000089808*thetadot4*cos(2.0*t5)*sin(2.0*t4) + 0.000089808*thetadot5*cos(2.0*t4)*sin(2.0*t5) + 0.010268*thetadot5*cos(t3)*cos(t4)*cos(t5) - 0.010268*thetadot3*cos(t4)*sin(t3)*sin(t5) - 0.010268*thetadot4*cos(t3)*sin(t4)*sin(t5),                                                                                                                                                                                                                                                                                                                                                                                                                                                                                                                                                                                                                                                                                                                                                                                                                                                                                                                                                                                                                                                                                                                                                                                                                                                                                                                                                                                                                                                                                                                                                                                                                                                                                                                                                                                                                                                                                                                                                                                                                                                                                                                                                                                                                                                                                                                                                                                                                                                                                                                                                                                                                                                                                                                                                                                                                                                        4.3855*thetadot2*cos(t3) - 0.000089808*thetadot5*sin(2.0*t5) - 0.0020898*thetadot4*sin(2.0*t4) + 2.1928*thetadot3*cos(t3) - 0.011148*thetadot5*sin(t5) + 0.010268*thetadot2*cos(t3)*cos(t5) + 0.0051341*thetadot3*cos(t3)*cos(t5) - 0.010268*thetadot5*sin(t3)*sin(t5) + 0.000089808*thetadot4*cos(2.0*t5)*sin(2.0*t4) + 0.000089808*thetadot5*cos(2.0*t4)*sin(2.0*t5) + 0.010268*thetadot5*cos(t3)*cos(t4)*cos(t5) - 0.010268*thetadot2*cos(t4)*sin(t3)*sin(t5) - 0.0051341*thetadot3*cos(t4)*sin(t3)*sin(t5) - 0.010268*thetadot4*cos(t3)*sin(t4)*sin(t5),                                                                                                                                                                                                                                                                                                                                                                                                                                                                                                                                                                                                                                                                                                                                                                                                                                                                                                                                                                                                                                                                                                                                                                                                                                                                                                                                                                     0.011*thetadot1*sin(t2)*sin(t3) - 0.0021796*thetadot3*sin(2.0*t4) - 0.001*thetadot4*cos(t4) - 0.011*thetadot1*cos(t2)*cos(t3) - 0.0055741*thetadot4*cos(t4)*sin(t5) - 0.011148*thetadot5*cos(t5)*sin(t4) - 0.0021796*thetadot2*sin(2.0*t4) - 0.00035923*thetadot5*cos(t5)^2*sin(t4) - 0.002*thetadot1*cos(t2)*cos(t4)*sin(t3) - 0.002*thetadot1*cos(t3)*cos(t4)*sin(t2) - 0.010268*thetadot1*cos(t2)*cos(t4)*sin(t5) - 0.00017962*thetadot4*cos(t4)*cos(t5)*sin(t5) - 0.010268*thetadot2*cos(t3)*sin(t4)*sin(t5) - 0.010268*thetadot3*cos(t3)*sin(t4)*sin(t5) - 0.0051341*thetadot4*cos(t4)*sin(t3)*sin(t5) - 0.010268*thetadot5*cos(t5)*sin(t3)*sin(t4) - 0.0043592*thetadot1*cos(t2)*cos(t3)*cos(t4)^2 + 0.00035923*thetadot2*cos(t4)*cos(t5)^2*sin(t4) + 0.00035923*thetadot3*cos(t4)*cos(t5)^2*sin(t4) + 0.0043592*thetadot1*cos(t4)^2*sin(t2)*sin(t3) - 0.00035923*thetadot1*cos(t4)^2*cos(t5)^2*sin(t2)*sin(t3) - 0.011148*thetadot1*cos(t2)*cos(t4)*sin(t3)*sin(t5) - 0.011148*thetadot1*cos(t3)*cos(t4)*sin(t2)*sin(t5) + 0.00035923*thetadot1*cos(t2)*cos(t3)*cos(t4)^2*cos(t5)^2 - 0.00035923*thetadot1*cos(t2)*cos(t4)*cos(t5)*sin(t3)*sin(t5) - 0.00035923*thetadot1*cos(t3)*cos(t4)*cos(t5)*sin(t2)*sin(t5),                                                                                                                                                                                                                                                                                                                                                                                                                                                                                                                                                                                                                                                                                                                                                                                                                                                                                                                                                                                                                                                                                                                                                                                                                                                                                                                                                    0.0051341*thetadot5*cos(t3)*cos(t5) - 0.00017962*thetadot3*sin(2.0*t5) - 0.011148*thetadot2*sin(t5) - 0.011148*thetadot3*sin(t5) - 0.00017962*thetadot2*sin(2.0*t5) - 0.011148*thetadot4*cos(t5)*sin(t4) - 0.0055741*thetadot5*cos(t4)*sin(t5) - 0.010268*thetadot2*sin(t3)*sin(t5) - 0.010268*thetadot3*sin(t3)*sin(t5) - 0.00035923*thetadot4*cos(t5)^2*sin(t4) + 0.010268*thetadot2*cos(t3)*cos(t4)*cos(t5) + 0.010268*thetadot3*cos(t3)*cos(t4)*cos(t5) - 0.010268*thetadot1*cos(t2)*cos(t5)*sin(t4) - 0.010268*thetadot4*cos(t5)*sin(t3)*sin(t4) - 0.0051341*thetadot5*cos(t4)*sin(t3)*sin(t5) + 0.00035923*thetadot2*cos(t4)^2*cos(t5)*sin(t5) + 0.00035923*thetadot3*cos(t4)^2*cos(t5)*sin(t5) - 0.011148*thetadot1*cos(t2)*cos(t5)*sin(t3)*sin(t4) - 0.011148*thetadot1*cos(t3)*cos(t5)*sin(t2)*sin(t4) - 0.00035923*thetadot1*cos(t2)*cos(t5)^2*sin(t3)*sin(t4) - 0.00035923*thetadot1*cos(t3)*cos(t5)^2*sin(t2)*sin(t4) - 0.00035923*thetadot1*cos(t2)*cos(t3)*cos(t4)*cos(t5)*sin(t4)*sin(t5) + 0.00035923*thetadot1*cos(t4)*cos(t5)*sin(t2)*sin(t3)*sin(t4)*sin(t5), 0;
                                                                                                                                                                                                                                                                                                                                                                                                                                                                                                                                                                                                                                                                                                                                                                                                                                                                                                                                                                                                                                                                                                                                                                                                                                                                                                                                                                                                                                                                                                                                                                                                                                                                                                                                                                                                                                                                                                                                                                                                                                                                  1.0964*thetadot1*cos(2.0*t2)*cos(t3) - 1.0964*thetadot1*cos(t3) - 1.0964*thetadot1*sin(2.0*t2)*sin(t3) - 0.002567*thetadot1*cos(t3)*cos(t5) - 0.01309*thetadot4*cos(t2)*cos(t3) + 0.01309*thetadot4*sin(t2)*sin(t3) + 0.83898*thetadot1*cos(2.0*t2)*sin(2.0*t3) + 0.83898*thetadot1*cos(2.0*t3)*sin(2.0*t2) - 0.002567*thetadot1*sin(2.0*t2)*cos(t5)*sin(t3) + 0.0020898*thetadot4*cos(2.0*t4)*sin(t2)*sin(t3) - 0.000089808*thetadot4*cos(2.0*t5)*sin(t2)*sin(t3) - 0.00052245*thetadot1*cos(2.0*t2)*cos(2.0*t4)*sin(2.0*t3) - 0.00052245*thetadot1*cos(2.0*t3)*cos(2.0*t4)*sin(2.0*t2) + 0.000067356*thetadot1*cos(2.0*t2)*cos(2.0*t5)*sin(2.0*t3) + 0.000067356*thetadot1*cos(2.0*t3)*cos(2.0*t5)*sin(2.0*t2) - 0.002*thetadot4*cos(t2)*cos(t4)*sin(t3) - 0.002*thetadot4*cos(t3)*cos(t4)*sin(t2) + 0.002567*thetadot1*cos(t4)*sin(t3)*sin(t5) - 0.00017962*thetadot5*cos(t2)*sin(t3)*sin(t4) - 0.00017962*thetadot5*cos(t3)*sin(t2)*sin(t4) + 0.001*thetadot1*cos(2.0*t2)*cos(2.0*t3)*cos(t4) + 0.0055741*thetadot1*cos(2.0*t2)*sin(2.0*t3)*cos(t5) + 0.0055741*thetadot1*cos(2.0*t3)*sin(2.0*t2)*cos(t5) - 0.001*thetadot1*sin(2.0*t2)*sin(2.0*t3)*cos(t4) + 0.002567*thetadot1*cos(2.0*t2)*cos(t3)*cos(t5) - 0.0020898*thetadot4*cos(2.0*t4)*cos(t2)*cos(t3) + 0.000089808*thetadot4*cos(2.0*t5)*cos(t2)*cos(t3) + 0.000089808*thetadot1*cos(2.0*t2)*cos(2.0*t3)*sin(2.0*t5)*cos(t4) - 0.000089808*thetadot1*sin(2.0*t2)*sin(2.0*t3)*sin(2.0*t5)*cos(t4) - 0.011148*thetadot4*cos(t2)*cos(t4)*sin(t3)*sin(t5) - 0.011148*thetadot4*cos(t3)*cos(t4)*sin(t2)*sin(t5) - 0.011148*thetadot5*cos(t2)*cos(t5)*sin(t3)*sin(t4) - 0.011148*thetadot5*cos(t3)*cos(t5)*sin(t2)*sin(t4) + 0.000089808*thetadot4*cos(2.0*t4)*cos(2.0*t5)*cos(t2)*cos(t3) + 0.0055741*thetadot1*cos(2.0*t2)*cos(2.0*t3)*cos(t4)*sin(t5) - 0.000089808*thetadot4*cos(2.0*t4)*cos(2.0*t5)*sin(t2)*sin(t3) - 0.000089808*thetadot5*sin(2.0*t4)*sin(2.0*t5)*cos(t2)*cos(t3) - 0.0055741*thetadot1*sin(2.0*t2)*sin(2.0*t3)*cos(t4)*sin(t5) + 0.000089808*thetadot5*sin(2.0*t4)*sin(2.0*t5)*sin(t2)*sin(t3) + 0.000022452*thetadot1*cos(2.0*t2)*cos(2.0*t4)*cos(2.0*t5)*sin(2.0*t3) + 0.000022452*thetadot1*cos(2.0*t3)*cos(2.0*t4)*cos(2.0*t5)*sin(2.0*t2) - 0.002567*thetadot1*cos(2.0*t2)*cos(t4)*sin(t3)*sin(t5) - 0.002567*thetadot1*sin(2.0*t2)*cos(t3)*cos(t4)*sin(t5) - 0.00017962*thetadot4*sin(2.0*t5)*cos(t2)*cos(t4)*sin(t3) - 0.00017962*thetadot4*sin(2.0*t5)*cos(t3)*cos(t4)*sin(t2) - 0.00017962*thetadot5*cos(2.0*t5)*cos(t2)*sin(t3)*sin(t4) - 0.00017962*thetadot5*cos(2.0*t5)*cos(t3)*sin(t2)*sin(t4),                                                                                                                                                                                                                                                                                                                                                                                                                                                                                                                                                                                                                                                                                                                                                                                                                                                                                                                                                                                                                                                                                                                                                                                                                                                                                                                                                                                                                                                                                                                                                                                                                                                                                                                                                                                                                                                                                                                                                                                                                                                                                                                                                                                                                                                                                                                                                                                                                                                                                                                                                                                                                                                                                                                                                                                                                                                                                                                                                                                                                                                                                          0.000089808*thetadot4*cos(2.0*t5)*sin(2.0*t4) - 0.000089808*thetadot5*sin(2.0*t5) - 2.1928*thetadot2*cos(t3) - 0.011148*thetadot5*sin(t5) - 0.0051341*thetadot2*cos(t3)*cos(t5) - 0.0020898*thetadot4*sin(2.0*t4) + 0.000089808*thetadot5*cos(2.0*t4)*sin(2.0*t5) + 0.0051341*thetadot2*cos(t4)*sin(t3)*sin(t5),                                                                                                                                                                                                                                                                                                                                                                                                                                                                                                                                                                                                                                                                                                                                                                                                                                                                                                                                                                                                                                                                                                                                                                                                                                                                                                                                                                                                                                                                                                                                                                                                                                                                                                                                                                                                                                                                                                                                                                                                                                                                                                                                                                                                                                                                                                                                                                                                                                                                                                                                                                                                                                                                                                                                                                                                                                                                                                                                                                                                                                                                                                                                                                                                                   0.000089808*thetadot4*cos(2.0*t5)*sin(2.0*t4) - 0.000089808*thetadot5*sin(2.0*t5) - 0.011148*thetadot5*sin(t5) - 0.0020898*thetadot4*sin(2.0*t4) + 0.000089808*thetadot5*cos(2.0*t4)*sin(2.0*t5),                                                                                                                                                                                                                                                                                                                                                                                                                                                                                                                                                                                                                                                                                                                                                                                                                                                                                                                                                                                                                                                                                                                                                                                                                                                                                                                                                                                                                                                                                                                                                                                                       0.011*thetadot1*sin(t2)*sin(t3) - 0.0021796*thetadot3*sin(2.0*t4) - 0.001*thetadot4*cos(t4) - 0.011*thetadot1*cos(t2)*cos(t3) - 0.0055741*thetadot4*cos(t4)*sin(t5) - 0.011148*thetadot5*cos(t5)*sin(t4) - 0.0021796*thetadot2*sin(2.0*t4) - 0.00035923*thetadot5*cos(t5)^2*sin(t4) - 0.002*thetadot1*cos(t2)*cos(t4)*sin(t3) - 0.002*thetadot1*cos(t3)*cos(t4)*sin(t2) - 0.00017962*thetadot4*cos(t4)*cos(t5)*sin(t5) - 0.0043592*thetadot1*cos(t2)*cos(t3)*cos(t4)^2 + 0.00035923*thetadot2*cos(t4)*cos(t5)^2*sin(t4) + 0.00035923*thetadot3*cos(t4)*cos(t5)^2*sin(t4) + 0.0043592*thetadot1*cos(t4)^2*sin(t2)*sin(t3) - 0.00035923*thetadot1*cos(t4)^2*cos(t5)^2*sin(t2)*sin(t3) - 0.011148*thetadot1*cos(t2)*cos(t4)*sin(t3)*sin(t5) - 0.011148*thetadot1*cos(t3)*cos(t4)*sin(t2)*sin(t5) + 0.00035923*thetadot1*cos(t2)*cos(t3)*cos(t4)^2*cos(t5)^2 - 0.00035923*thetadot1*cos(t2)*cos(t4)*cos(t5)*sin(t3)*sin(t5) - 0.00035923*thetadot1*cos(t3)*cos(t4)*cos(t5)*sin(t2)*sin(t5),                                                                                                                                                                                                                                                                                                                                                                                                                                                                                                                                                                                                                                                                                                                                                                                                                                                                                                                                                                                                                                                                                                                                                                                                                                                                                                                                                                                                                                                                                                                                                                                                                                                                                                      0.00035923*thetadot2*cos(t4)^2*cos(t5)*sin(t5) - 0.00017962*thetadot3*sin(2.0*t5) - 0.011148*thetadot2*sin(t5) - 0.011148*thetadot3*sin(t5) - 0.011148*thetadot4*cos(t5)*sin(t4) - 0.0055741*thetadot5*cos(t4)*sin(t5) - 0.00035923*thetadot4*cos(t5)^2*sin(t4) - 0.00017962*thetadot2*sin(2.0*t5) + 0.00035923*thetadot3*cos(t4)^2*cos(t5)*sin(t5) - 0.011148*thetadot1*cos(t2)*cos(t5)*sin(t3)*sin(t4) - 0.011148*thetadot1*cos(t3)*cos(t5)*sin(t2)*sin(t4) - 0.00035923*thetadot1*cos(t2)*cos(t5)^2*sin(t3)*sin(t4) - 0.00035923*thetadot1*cos(t3)*cos(t5)^2*sin(t2)*sin(t4) - 0.00035923*thetadot1*cos(t2)*cos(t3)*cos(t4)*cos(t5)*sin(t4)*sin(t5) + 0.00035923*thetadot1*cos(t4)*cos(t5)*sin(t2)*sin(t3)*sin(t4)*sin(t5), 0;
                                                                                                                                                                                                                                                                                                                                                                                                                                                                                                                                                                                                                                                                                                                                                                                                                                                                                                                                                                                                                                                                                                                                                                                                                                                                                                                                                                                                                                                                                                                                                                                                                                                                                                                                                                                                                                                                                                        0.01309*thetadot2*cos(t2)*cos(t3) - 0.00052245*thetadot1*sin(2.0*t4) + 0.01309*thetadot3*cos(t2)*cos(t3) - 0.01309*thetadot2*sin(t2)*sin(t3) - 0.01309*thetadot3*sin(t2)*sin(t3) + 0.000022452*thetadot1*cos(2.0*t5)*sin(2.0*t4) - 0.0020898*thetadot2*cos(2.0*t4)*sin(t2)*sin(t3) + 0.000089808*thetadot2*cos(2.0*t5)*sin(t2)*sin(t3) - 0.0020898*thetadot3*cos(2.0*t4)*sin(t2)*sin(t3) + 0.000089808*thetadot3*cos(2.0*t5)*sin(t2)*sin(t3) + 0.00017962*thetadot5*sin(2.0*t5)*cos(t2)*sin(t3) + 0.00017962*thetadot5*sin(2.0*t5)*cos(t3)*sin(t2) - 0.00052245*thetadot1*cos(2.0*t2)*cos(2.0*t3)*sin(2.0*t4) + 0.00017962*thetadot5*cos(t2)*cos(t3)*cos(t4) + 0.00052245*thetadot1*sin(2.0*t2)*sin(2.0*t3)*sin(2.0*t4) + 0.002*thetadot2*cos(t2)*cos(t4)*sin(t3) + 0.002*thetadot2*cos(t3)*cos(t4)*sin(t2) + 0.002*thetadot3*cos(t2)*cos(t4)*sin(t3) + 0.002*thetadot3*cos(t3)*cos(t4)*sin(t2) + 0.010268*thetadot2*cos(t2)*cos(t4)*sin(t5) + 0.002567*thetadot1*cos(t3)*sin(t4)*sin(t5) - 0.00017962*thetadot5*cos(t4)*sin(t2)*sin(t3) - 0.0005*thetadot1*cos(2.0*t2)*sin(2.0*t3)*sin(t4) - 0.0005*thetadot1*cos(2.0*t3)*sin(2.0*t2)*sin(t4) + 0.0020898*thetadot2*cos(2.0*t4)*cos(t2)*cos(t3) - 0.000089808*thetadot2*cos(2.0*t5)*cos(t2)*cos(t3) + 0.0020898*thetadot3*cos(2.0*t4)*cos(t2)*cos(t3) - 0.000089808*thetadot3*cos(2.0*t5)*cos(t2)*cos(t3) + 0.002567*thetadot1*sin(2.0*t2)*sin(t3)*sin(t4)*sin(t5) - 0.000044904*thetadot1*cos(2.0*t2)*sin(2.0*t3)*sin(2.0*t5)*sin(t4) - 0.000044904*thetadot1*cos(2.0*t3)*sin(2.0*t2)*sin(2.0*t5)*sin(t4) + 0.011148*thetadot2*cos(t2)*cos(t4)*sin(t3)*sin(t5) + 0.011148*thetadot2*cos(t3)*cos(t4)*sin(t2)*sin(t5) + 0.011148*thetadot3*cos(t2)*cos(t4)*sin(t3)*sin(t5) + 0.011148*thetadot3*cos(t3)*cos(t4)*sin(t2)*sin(t5) - 0.000089808*thetadot2*cos(2.0*t4)*cos(2.0*t5)*cos(t2)*cos(t3) - 0.000089808*thetadot3*cos(2.0*t4)*cos(2.0*t5)*cos(t2)*cos(t3) + 0.000089808*thetadot2*cos(2.0*t4)*cos(2.0*t5)*sin(t2)*sin(t3) + 0.000089808*thetadot3*cos(2.0*t4)*cos(2.0*t5)*sin(t2)*sin(t3) - 0.0027871*thetadot1*cos(2.0*t2)*sin(2.0*t3)*sin(t4)*sin(t5) - 0.0027871*thetadot1*cos(2.0*t3)*sin(2.0*t2)*sin(t4)*sin(t5) + 0.000022452*thetadot1*cos(2.0*t2)*cos(2.0*t3)*cos(2.0*t5)*sin(2.0*t4) - 0.00017962*thetadot5*cos(2.0*t5)*cos(t2)*cos(t3)*cos(t4) - 0.000022452*thetadot1*cos(2.0*t5)*sin(2.0*t2)*sin(2.0*t3)*sin(2.0*t4) - 0.002567*thetadot1*cos(2.0*t2)*cos(t3)*sin(t4)*sin(t5) + 0.00017962*thetadot2*sin(2.0*t5)*cos(t2)*cos(t4)*sin(t3) + 0.00017962*thetadot2*sin(2.0*t5)*cos(t3)*cos(t4)*sin(t2) + 0.00017962*thetadot3*sin(2.0*t5)*cos(t2)*cos(t4)*sin(t3) + 0.00017962*thetadot3*sin(2.0*t5)*cos(t3)*cos(t4)*sin(t2) + 0.00017962*thetadot5*cos(2.0*t5)*cos(t4)*sin(t2)*sin(t3),                                                                                                                                                                                                                                                                                                                                                                                                                                                                                                                                                                                                                                                                                                                                                                                                                                                                                                                                                                                                                                                                                                                                                                                                                                                                                                                                                                                                                                                                                                                                                                                                                                                                                                                                                                                                                                                                                                                                                                                                                                                                                                                                                                                                                                                                                                                                                                                                                                             0.0010898*thetadot2*sin(2.0*t4) + 0.0021796*thetadot3*sin(2.0*t4) + 0.00035923*thetadot5*sin(t4) + 0.011*thetadot1*cos(t2)*cos(t3) - 0.011*thetadot1*sin(t2)*sin(t3) - 0.00035923*thetadot5*cos(t5)^2*sin(t4) + 0.002*thetadot1*cos(t2)*cos(t4)*sin(t3) + 0.002*thetadot1*cos(t3)*cos(t4)*sin(t2) + 0.010268*thetadot1*cos(t2)*cos(t4)*sin(t5) + 0.0051341*thetadot2*cos(t3)*sin(t4)*sin(t5) + 0.0043592*thetadot1*cos(t2)*cos(t3)*cos(t4)^2 - 0.00017962*thetadot2*cos(t4)*cos(t5)^2*sin(t4) - 0.00035923*thetadot3*cos(t4)*cos(t5)^2*sin(t4) - 0.0043592*thetadot1*cos(t4)^2*sin(t2)*sin(t3) + 0.00035923*thetadot1*cos(t4)^2*cos(t5)^2*sin(t2)*sin(t3) + 0.011148*thetadot1*cos(t2)*cos(t4)*sin(t3)*sin(t5) + 0.011148*thetadot1*cos(t3)*cos(t4)*sin(t2)*sin(t5) - 0.00035923*thetadot1*cos(t2)*cos(t3)*cos(t4)^2*cos(t5)^2 + 0.00035923*thetadot1*cos(t2)*cos(t4)*cos(t5)*sin(t3)*sin(t5) + 0.00035923*thetadot1*cos(t3)*cos(t4)*cos(t5)*sin(t2)*sin(t5),                                                                                                                                                                                                                                                                                                                                                                                                                                                                                                                                                                                                                                                                                                                                                                                                                                                                                                                                                                                                                                                                                                                                                                                                                                                                                                                                                                                                                                                                                                                                                                                                                                                                                                                                                                                                                                                                                                                                                                                                                                                                                                                                                                                                                                                                                                                                                                                                                                                                                                                                                  0.0021796*thetadot2*sin(2.0*t4) + 0.0010898*thetadot3*sin(2.0*t4) + 0.00035923*thetadot5*sin(t4) + 0.011*thetadot1*cos(t2)*cos(t3) - 0.011*thetadot1*sin(t2)*sin(t3) - 0.00035923*thetadot5*cos(t5)^2*sin(t4) + 0.002*thetadot1*cos(t2)*cos(t4)*sin(t3) + 0.002*thetadot1*cos(t3)*cos(t4)*sin(t2) + 0.0043592*thetadot1*cos(t2)*cos(t3)*cos(t4)^2 - 0.00035923*thetadot2*cos(t4)*cos(t5)^2*sin(t4) - 0.00017962*thetadot3*cos(t4)*cos(t5)^2*sin(t4) - 0.0043592*thetadot1*cos(t4)^2*sin(t2)*sin(t3) + 0.00035923*thetadot1*cos(t4)^2*cos(t5)^2*sin(t2)*sin(t3) + 0.011148*thetadot1*cos(t2)*cos(t4)*sin(t3)*sin(t5) + 0.011148*thetadot1*cos(t3)*cos(t4)*sin(t2)*sin(t5) - 0.00035923*thetadot1*cos(t2)*cos(t3)*cos(t4)^2*cos(t5)^2 + 0.00035923*thetadot1*cos(t2)*cos(t4)*cos(t5)*sin(t3)*sin(t5) + 0.00035923*thetadot1*cos(t3)*cos(t4)*cos(t5)*sin(t2)*sin(t5),                                                                                                                                                                                                                                                                                                                                                                                                                                                                                                                                                                                                                                                                                                                                                                                                                                                                                                                                                                                                                                                                                                                                                                                                                                                                                                                                                                                                                                                                                                                                                                                                                                                                                                                                                                                                                                                                                                                                                                                                                                                                                                                                                                                                                                                                                                                                                                                                                                                                                                                                                             0.00017962*thetadot5*sin(2.0*t5),                                                                                                                                                                                                                                                                                                                                                                                                                                                                                                                                                                                                                                                                                                                                                                                                                                                                                                                                                                                                                                                                                                                                                                                                                                                                                                                                                                                                                                                                                                                                                                                                                                                                                                                                                                                                                                                                                                                                                                                                                                                                                                                                                                                                               sin(t5)*(0.00035923*thetadot4*cos(t5) + 0.00035923*thetadot1*sin(t2 + t3)*cos(t5) + 0.00035923*thetadot2*sin(t4)*sin(t5) + 0.00035923*thetadot3*sin(t4)*sin(t5) + 0.00035923*thetadot1*cos(t2 + t3)*cos(t4)*sin(t5)), 0;
                                                                                                                                                                                                                                                                                                                                                                                                                                                                                                                                                                                                                                                                                                                                                                                                                                                                                                                                                                                                                                                                                                                                                                                                                                                                                                                                                                                                                                                                                                                                                                                                                                                                                                                                                                                                                                                                                                                                                                                                                                                                                                                                                                                                                                                                              0.0027871*thetadot1*sin(t5) - 0.000022452*thetadot1*sin(2.0*t5) + 0.002567*thetadot1*sin(t3)*sin(t5) + 0.000022452*thetadot1*cos(2.0*t4)*sin(2.0*t5) - 0.002567*thetadot1*cos(2.0*t2)*sin(t3)*sin(t5) - 0.002567*thetadot1*sin(2.0*t2)*cos(t3)*sin(t5) - 0.00017962*thetadot4*sin(2.0*t5)*cos(t2)*sin(t3) - 0.00017962*thetadot4*sin(2.0*t5)*cos(t3)*sin(t2) + 0.000067356*thetadot1*cos(2.0*t2)*cos(2.0*t3)*sin(2.0*t5) - 0.002567*thetadot1*cos(t3)*cos(t4)*cos(t5) - 0.00017962*thetadot4*cos(t2)*cos(t3)*cos(t4) - 0.000067356*thetadot1*sin(2.0*t2)*sin(2.0*t3)*sin(2.0*t5) + 0.010268*thetadot2*cos(t2)*cos(t5)*sin(t4) + 0.00017962*thetadot2*cos(t2)*sin(t3)*sin(t4) + 0.00017962*thetadot2*cos(t3)*sin(t2)*sin(t4) + 0.00017962*thetadot3*cos(t2)*sin(t3)*sin(t4) + 0.00017962*thetadot3*cos(t3)*sin(t2)*sin(t4) + 0.00017962*thetadot4*cos(t4)*sin(t2)*sin(t3) + 0.0027871*thetadot1*cos(2.0*t2)*cos(2.0*t3)*sin(t5) - 0.0027871*thetadot1*sin(2.0*t2)*sin(2.0*t3)*sin(t5) + 0.000089808*thetadot1*cos(2.0*t2)*cos(2.0*t5)*sin(2.0*t3)*cos(t4) + 0.000089808*thetadot1*cos(2.0*t3)*cos(2.0*t5)*sin(2.0*t2)*cos(t4) + 0.011148*thetadot2*cos(t2)*cos(t5)*sin(t3)*sin(t4) + 0.011148*thetadot2*cos(t3)*cos(t5)*sin(t2)*sin(t4) + 0.011148*thetadot3*cos(t2)*cos(t5)*sin(t3)*sin(t4) + 0.011148*thetadot3*cos(t3)*cos(t5)*sin(t2)*sin(t4) + 0.0027871*thetadot1*cos(2.0*t2)*sin(2.0*t3)*cos(t4)*cos(t5) + 0.0027871*thetadot1*cos(2.0*t3)*sin(2.0*t2)*cos(t4)*cos(t5) + 0.000089808*thetadot2*sin(2.0*t4)*sin(2.0*t5)*cos(t2)*cos(t3) + 0.000089808*thetadot3*sin(2.0*t4)*sin(2.0*t5)*cos(t2)*cos(t3) - 0.000089808*thetadot2*sin(2.0*t4)*sin(2.0*t5)*sin(t2)*sin(t3) - 0.000089808*thetadot3*sin(2.0*t4)*sin(2.0*t5)*sin(t2)*sin(t3) + 0.000022452*thetadot1*cos(2.0*t2)*cos(2.0*t3)*cos(2.0*t4)*sin(2.0*t5) + 0.002567*thetadot1*cos(2.0*t2)*cos(t3)*cos(t4)*cos(t5) + 0.00017962*thetadot4*cos(2.0*t5)*cos(t2)*cos(t3)*cos(t4) - 0.000022452*thetadot1*cos(2.0*t4)*sin(2.0*t2)*sin(2.0*t3)*sin(2.0*t5) - 0.002567*thetadot1*sin(2.0*t2)*cos(t4)*cos(t5)*sin(t3) + 0.00017962*thetadot2*cos(2.0*t5)*cos(t2)*sin(t3)*sin(t4) + 0.00017962*thetadot2*cos(2.0*t5)*cos(t3)*sin(t2)*sin(t4) + 0.00017962*thetadot3*cos(2.0*t5)*cos(t2)*sin(t3)*sin(t4) + 0.00017962*thetadot3*cos(2.0*t5)*cos(t3)*sin(t2)*sin(t4) - 0.00017962*thetadot4*cos(2.0*t5)*cos(t4)*sin(t2)*sin(t3),                                                                                                                                                                                                                                                                                                                                                                                                                                                                                                                                                                                                                                                                                                                                                                                                                                                                                                                                                                                                                                                                                                                                                                                                                                                                                                                                                                                                                                                                                                                                                                                                                                                                                                                                                                                                                                                                                                                                                                                                                                                                                                                                                                                                                                                                                                                                                                                                                                                                                                                                                                                     0.000089808*thetadot2*sin(2.0*t5) + 0.00017962*thetadot3*sin(2.0*t5) + 0.0055741*thetadot2*sin(t5) + 0.011148*thetadot3*sin(t5) - 0.00035923*thetadot4*sin(t4) + 0.0051341*thetadot2*sin(t3)*sin(t5) + 0.00035923*thetadot4*cos(t5)^2*sin(t4) - 0.0051341*thetadot2*cos(t3)*cos(t4)*cos(t5) + 0.010268*thetadot1*cos(t2)*cos(t5)*sin(t4) - 0.00017962*thetadot2*cos(t4)^2*cos(t5)*sin(t5) - 0.00035923*thetadot3*cos(t4)^2*cos(t5)*sin(t5) + 0.011148*thetadot1*cos(t2)*cos(t5)*sin(t3)*sin(t4) + 0.011148*thetadot1*cos(t3)*cos(t5)*sin(t2)*sin(t4) + 0.00035923*thetadot1*cos(t2)*cos(t5)^2*sin(t3)*sin(t4) + 0.00035923*thetadot1*cos(t3)*cos(t5)^2*sin(t2)*sin(t4) + 0.00035923*thetadot1*cos(t2)*cos(t3)*cos(t4)*cos(t5)*sin(t4)*sin(t5) - 0.00035923*thetadot1*cos(t4)*cos(t5)*sin(t2)*sin(t3)*sin(t4)*sin(t5),                                                                                                                                                                                                                                                                                                                                                                                                                                                                                                                                                                                                                                                                                                                                                                                                                                                                                                                                                                                                                                                                                                                                                                                                                                                                                                                                                                                                                                                                                                                                                                                                                                                                                                                                                                                                                                                                                                                                                                                                                                                                                                                                                                                                                                                                                                                                                                                                                                                                                                                                                                                                                                                                                                                                0.00017962*thetadot2*sin(2.0*t5) + 0.000089808*thetadot3*sin(2.0*t5) + 0.011148*thetadot2*sin(t5) + 0.0055741*thetadot3*sin(t5) - 0.00035923*thetadot4*sin(t4) + 0.00035923*thetadot4*cos(t5)^2*sin(t4) - 0.00035923*thetadot2*cos(t4)^2*cos(t5)*sin(t5) - 0.00017962*thetadot3*cos(t4)^2*cos(t5)*sin(t5) + 0.011148*thetadot1*cos(t2)*cos(t5)*sin(t3)*sin(t4) + 0.011148*thetadot1*cos(t3)*cos(t5)*sin(t2)*sin(t4) + 0.00035923*thetadot1*cos(t2)*cos(t5)^2*sin(t3)*sin(t4) + 0.00035923*thetadot1*cos(t3)*cos(t5)^2*sin(t2)*sin(t4) + 0.00035923*thetadot1*cos(t2)*cos(t3)*cos(t4)*cos(t5)*sin(t4)*sin(t5) - 0.00035923*thetadot1*cos(t4)*cos(t5)*sin(t2)*sin(t3)*sin(t4)*sin(t5),                                                                                                                                                                                                                                                                                                                                                                                                                                                                                                                                                                                                                                                                                                                                                                                                                                                                                                                                                                                                                                                                                                                                                                                                                                                                                                                                                                                                                                                                                                                                                                                                                                                                                                                                                                                                                                                                                                                                                                                                                                                                              0.00017962*thetadot2*cos(2.0*t5)*sin(t4) - 0.00017962*thetadot2*sin(t4) - 0.00017962*thetadot3*sin(t4) - 0.000089808*thetadot4*sin(2.0*t5) + 0.00017962*thetadot3*cos(2.0*t5)*sin(t4) - 0.00017962*thetadot1*sin(2.0*t5)*cos(t2)*sin(t3) - 0.00017962*thetadot1*sin(2.0*t5)*cos(t3)*sin(t2) - 0.00017962*thetadot1*cos(t2)*cos(t3)*cos(t4) + 0.00017962*thetadot1*cos(t4)*sin(t2)*sin(t3) + 0.00017962*thetadot1*cos(2.0*t5)*cos(t2)*cos(t3)*cos(t4) - 0.00017962*thetadot1*cos(2.0*t5)*cos(t4)*sin(t2)*sin(t3),                                                                                                                                                                                                                                                                                                                                                                                                                                                                                                                                                                                                                                                                                                                                                                                                                                                                                                                                                                                                                                                                                                                                                                                                                                                                                                                                                                                                                                                                                                                                                                                                                                                                                                                                                                                                                                                                                                                                                                                                                                                                                                                                                                                                                                                                                                                                                                                                                                  0, 0;
                                                                                                                                                                                                                                                                                                                                                                                                                                                                                                                                                                                                                                                                                                                                                                                                                                                                                                                                                                                                                                                                                                                                                                                                                                                                                                                                                                                                                                                                                                                                                                                                                                                                                                                                                                                                                                                                                                                                                                                                                                                                                                                                                                                                                                                                                                                                                                                                                                                                                                                                                                                                                                                                                                                                                                                                                                                                                                                                                                                                                                                                                                                                                                                                                                                                                                                                                                                                                                                                                                                                                                                                                                                                                                                                                                                                                                                                                                                                                                                                                                                                                                                                                                                                                                                                                                                                                                                                                                                                                                                                                                                                                                                             0,                                                                                                                                                                                                                                                                                                                                                                                                                                                                                                                                                                                                                                                                                                                                                                                                                                                                                                                                                                                                                                                                                                                                                                                                                                                                                                                                                                                                                                                                                                                                                                                                                                                                                                                                                                                                                                                                                                                                                                                                                                                                                                                                                                                                                                                                                                                                                                                                                                                                                                                                                                                                                                                                                                                                                                                                                                                                                                                                                                                                                                                                                                                                                                                                                                                                                                                                                                                                        0,                                                                                                                                                                                                                                                                                                                                                                                                                                                                                                                                                                                                                                                                                                                                                                                                                                                                                                                                                                                                                                                                                                                                                                                                                                                                                                                                                                                                                                                                                                                                                                                                                                                                                                                                                                                                                                                                                                                                                                                                                                                                                                                                                                                                                                                                                                                                                                                                                                                                                                                                                                                                                                                                                                                                                                                                                                                                                                                                                                                                                                                                                                                                                                                                                                                                                                                                                                                                                  0,                                                                                                                                                                                                                                                                                                                                                                                                                                                                                                                                                                                                                                                                                                                                                                                                                                                                                                                                                                                                                                                                                                                                                                                                                                                                                                                                                                                                                                                                                                                                                                                                                                                                                                                                                                                                                                                                                                                                                                                                                                                                                                                                                                                                                                                                                                                                                                                                                                                                                                                                                                                            0,                                                                                                                                                                                                                                                                                                                                                                                                                                                                                                                                                                                                                                                                                                                                                                                                                                                                                                                                                                                                                                                                                                                                                                                                                                                                                                                                                                                                                                                                                                                                                                                                                                                                                                                                                                                                                                                                                                                                                                                                                                                                                                                                                                                                                                                                                                                                                                                                                                  0, 0];






 G=[                                                                                                                                                                                                                               0;
 3.1325*cos(t2)*cos(t3) - 16.138*sin(t2) - 3.1325*sin(t2)*sin(t3) - 0.0073344*cos(t5)*sin(t2)*sin(t3) + 0.0073344*cos(t2)*cos(t3)*cos(t5) - 0.0073344*cos(t2)*cos(t4)*sin(t3)*sin(t5) - 0.0073344*cos(t3)*cos(t4)*sin(t2)*sin(t5);
                  3.1325*cos(t2)*cos(t3) - 3.1325*sin(t2)*sin(t3) - 0.0073344*cos(t5)*sin(t2)*sin(t3) + 0.0073344*cos(t2)*cos(t3)*cos(t5) - 0.0073344*cos(t2)*cos(t4)*sin(t3)*sin(t5) - 0.0073344*cos(t3)*cos(t4)*sin(t2)*sin(t5);
                                                                                                                                                                                          -0.0073344*cos(t2 + t3)*sin(t4)*sin(t5);
                                                                    0.0073344*cos(t2)*cos(t3)*cos(t4)*cos(t5) - 0.0073344*cos(t3)*sin(t2)*sin(t5) - 0.0073344*cos(t2)*sin(t3)*sin(t5) - 0.0073344*cos(t4)*cos(t5)*sin(t2)*sin(t3);
                                                                                                                                                                                                                                0];





I_m=diag([0.1 0.1 0.1 0.1 0.1]);
B_m=diag([0.01 0.01 0.01 0.01 0.01]);
r=100;
q_ddot=inv(I_m+M(1:5,1:5)/r^2)*(U(1:5)-(B_m+C(1:5,1:5)/r)*tdot(1:5));%#ok


end
